simulink model "interpolation_cubique"  (R2017b)
settings: Solver=FixedStepDiscrete  StartTime=0.0  StopTime=1  RelTol=1e-3
model workspace (MAT data in the model file):
  bande_passante = 20000000
  binary_sample_time = 2.51968503937e-08
  display = [0 0 0 0 0 0 0 0 0 0 0 0 ... (40000 elements, 200x200)]
  nbr_pilote = 3
  nbr_sous_porteuse = 508
  nbr_total_canaux = 512
  nbr_zero = 1
  size_prefixe_cyclique = 3
  symbol_sample_time = 2.56e-05
  v = [0 0 0 0 0 0 0 0 0 0 0 0 ... (256 elements, 256x1)]
values from neighbouring files (symbols this model uses):
  interval_pilote = 150    [workspace.m]
undefined symbols (not defined in the file or in its folder): doppler
libraries: commchan3 x2, dspxfrm3 x2, dspindex x2, commdigbbndpm3 x2, commrandsrc3 x1, commsink2 x1
(part 2 of 2)

== matlab function interpolation_cubique/MATLAB Function1 ==
  data: u input; y output; nbr_zero parameter; nbr_total_canaux parameter; interval_pilote parameter; nbr_sous_porteuse parameter; nbr_pilote parameter
function y = fcn(u, nbr_zero, nbr_total_canaux, interval_pilote, nbr_sous_porteuse, nbr_pilote)


v3 = zeros(1,nbr_sous_porteuse);
v4 = zeros(1,nbr_sous_porteuse);
data_sous_porteuse = complex(v3,v4);

v1 = zeros(1,nbr_pilote);
v2 = zeros(1,nbr_pilote);
vecteur_pilote = complex(v1,v2);

l = interval_pilote;
l2 =fix(interval_pilote/2);
compteur_sous_porteuse = 1;
compteur_pilote = 1;


for k=fix(nbr_zero/2)+1:1:nbr_total_canaux-(fix(nbr_zero/2)+rem(nbr_zero,2))
    if l2 == 0
        l2 = l;
        vecteur_pilote(compteur_pilote) = u(k);
        compteur_pilote = compteur_pilote + 1;
    else
        data_sous_porteuse(compteur_sous_porteuse) = u(k);
        compteur_sous_porteuse = compteur_sous_porteuse + 1;
        l2 = l2 -1;
    end
end

x = 1:1:nbr_pilote;
xq = linspace(1,nbr_pilote, nbr_sous_porteuse);
interpolation_pilote = interp1(x,vecteur_pilote,xq,'pchip');
plot(x,vecteur_pilote,'o',xq,interpolation_pilote,':.');

for j = 1 :1: nbr_sous_porteuse 
    data_sous_porteuse(j) = data_sous_porteuse(j)./ interpolation_pilote(j);
end
 

y = data_sous_porteuse.';

== matlab function interpolation_cubique/MATLAB Function ==
  data: u input; y output; nbr_total_canaux parameter; nbr_zero parameter; interval_pilote parameter
function y = fcn(u, nbr_total_canaux, nbr_zero, interval_pilote)
i = interval_pilote; %Sélection du nombre de pilote 
n = nbr_total_canaux; %Nombre de sous-canaux
v1 = zeros(n,1);
v2 = zeros(n,1);
v = complex(v1,v2);
l = interval_pilote;
l2 = fix(interval_pilote/2);
u_compteur = 1;
l_compteur = 0;

for k=fix(nbr_zero/2)+1:1:nbr_total_canaux-(fix(nbr_zero/2)+rem(nbr_zero,2))
    if l2 == 0
        l2 = l;
        v(k) = complex(1);
        l_compteur = l_compteur + 1;
    else 
        v(k) = u(u_compteur);   
        l2 = l2 - 1;
        u_compteur = u_compteur + 1; 
    end
end
y = v;

== matlab function interpolation_cubique/MATLAB Function2 ==
  data: u input; y output
function y = fcn(u)

L = length(u);
somme = 0;
for k=1:1:L
    somme = somme + abs(u(k))^2;
end

somme = somme/L; 
        
disp(somme);

y = somme;
